simulink model "Drivetrain"  (R2013a)
settings: Solver=FixedStepDiscrete  StartTime=0.0  StopTime=10.0  FixedStep=.001  RelTol=1e-3
undefined symbols (not defined in the file or in its folder): power_lim, torque_lim
libraries: fl_lib x10, nesl_utility x6, sdl_lib x3, simulink x1
settings Model: Creator=noah  LastModifiedBy=ntfox
settings DataIOCC: SignalLoggingSaveFormat=ModelDataLogs
settings DebuggingCC: UnderspecifiedInitializationDetection=Simplified  MultiTaskDSMMsg=warning  MultiTaskCondExecSysMsg=none  StateNameClashWarn=none  StrictBusMsg=ErrorOnBusTreatedAsVector
settings RTWCC: IncludeERTFirstTime=on
settings GRTTargetCC: CodeReplacementLibrary=None  CPPClassGenCompliant=on

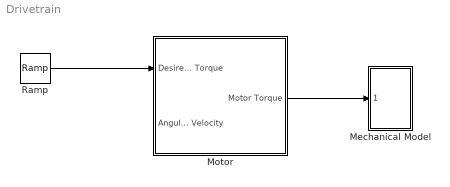
== system Drivetrain ==
  Mechanical Model : Subsystem
  Motor : Subsystem
  Ramp : simulink/Sources/Ramp  slope=1  start=0  X0=0
  wires:
  Motor/1(Motor Torque) -> Mechanical Model/1(Torque)
  Ramp/1 -> Motor/1(Desired Torque)

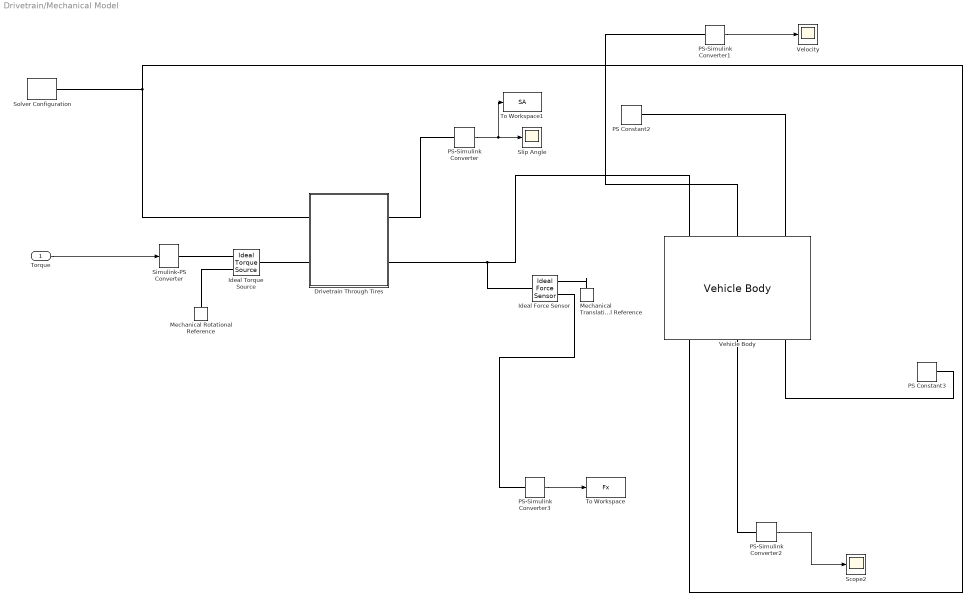
== system Drivetrain/Mechanical Model ==
  Torque : Inport
  Drivetrain Through Tires : Subsystem
  Ideal Force Sensor : fl_lib/Mechanical/Mechanical Sensors/Ideal Force Sensor  v_Log=off  f_Log=off  LocalVarNames=|v|f  LocalVarDescs=|v|f  LocalVarLogging=[0 0]
  Ideal Torque Source : fl_lib/Mechanical/Mechanical Sources/Ideal Torque Source  w_Log=off  t_Log=off  LocalVarNames=|w|t  LocalVarDescs=|w|t  LocalVarLogging=[0 0]
  Mechanical Rotational Reference : fl_lib/Mechanical/Rotational Elements/Mechanical Rotational Reference  t_Log=off  LocalVarNames=|t  LocalVarDescs=|t  LocalVarLogging=0
  Mechanical Translational Reference : fl_lib/Mechanical/Translational Elements/Mechanical Translational Reference  f_Log=off  LocalVarNames=|f  LocalVarDescs=|f  LocalVarLogging=0
  PS Constant2 : fl_lib/Physical Signals/Sources/PS Constant  constant=0  LocalVarLogging=[]
  PS Constant3 : fl_lib/Physical Signals/Sources/PS Constant  constant=0  LocalVarLogging=[]
  PS-Simulink Converter{,1..3} (4 alike) : nesl_utility/PS-Simulink Converter  PhysicalDomain=network_engine_domain  SubClassName=ps_output  LeftPortType=input  RightPortType=output  PseudoPeriodic=off  Frequencies=[]  Unit=1  AffineConversion=off
  Scope2 : Scope
      settings: SaveName=ScopeData2
  Simulink-PS Converter : nesl_utility/Simulink-PS Converter  PhysicalDomain=network_engine_domain  SubClassName=ps_input  LeftPortType=input  RightPortType=output  PseudoPeriodic=off  Frequencies=[]  NoiseDistribution=none  NoiseParameters=[]  Unit=1  AffineConversion=off  InputFiltering=off  SimscapeFilterOrder=1  InputFilterTimeConstant=0.001  UdotUserProvided=1
  Slip Angle : Scope
      settings: TimeRange=10  YMin=0  YMax=9000
  Solver Configuration : nesl_utility/Solver Configuration  PhysicalDomain=network_engine_domain  SubClassName=solver  LeftPortType=input  RightPortType=generic  Accelerate=off  Tones=[]  Harmonics=[]  SimulateNoise=off  Profile=off  UseLocalSampling=off  EnableSwitchedLinearOptims=on  FrequencyDomain=off  UseCCode=off  UseNewInitialization=off  DoDC=off  ResidualTolerance=1e-09  UseLocalSolver=off  LocalSolverChoice=NE_BACKWARD_EULER_ADVANCER  LocalSolverSampleTime=0.001  DoFixedCost=off  MaxNonlinIter=3  MaxModeIter=2  LinearAlgebra=Sparse  DelaysMemoryBudget=1024
  To Workspace : ToWorkspace  VariableName=Fx  SampleTime=-1  SaveFormat=Timeseries
  To Workspace1 : ToWorkspace  VariableName=SA  SampleTime=-1  SaveFormat=Timeseries
  Vehicle Body : sdl_lib/Tires & Vehicles/Vehicle Body  mass=300 kg  n_w=2  x_f=.8 m  x_r=.8 m  y_c=.2 m  area=3 m^2  Cd=0.4  v0=0 m/s  g=9.81 m/s^2  rho=1.18 kg/m^3  v_Log=off  f_Log=off  LocalVarNames=|v|f  LocalVarDescs=|v|f  LocalVarLogging=[0 0]
  Velocity : Scope
      settings: TimeRange=10  YMin=0  YMax=6
  wires:
  PS-Simulink Converter/1 -> To Workspace1/1, Slip Angle/1
  PS-Simulink Converter1/1 -> Velocity/1
  PS-Simulink Converter2/1 -> Scope2/1
  PS-Simulink Converter3/1 -> To Workspace/1
  Torque/1 -> Simulink-PS Converter/1
  connections:
  Simulink-PS Converter/RConn1 -- Ideal Torque Source/RConn1
  Mechanical Rotational Reference/LConn1 -- Ideal Torque Source/RConn2
  Drivetrain Through Tires/LConn2 -- Ideal Torque Source/LConn1
  PS-Simulink Converter/LConn1 -- Drivetrain Through Tires/RConn1
  Vehicle Body/RConn1 -- Drivetrain Through Tires/LConn1 -- Solver Configuration/RConn1
  Vehicle Body/RConn2 -- PS-Simulink Converter2/LConn1
  PS Constant2/RConn1 -- Vehicle Body/LConn3
  Vehicle Body/LConn2 -- PS-Simulink Converter1/LConn1
  PS Constant3/RConn1 -- Vehicle Body/RConn3
  Ideal Force Sensor/RConn2 -- PS-Simulink Converter3/LConn1
  Mechanical Translational Reference/LConn1 -- Ideal Force Sensor/RConn1
  Vehicle Body/LConn1 -- Ideal Force Sensor/LConn1 -- Drivetrain Through Tires/RConn2

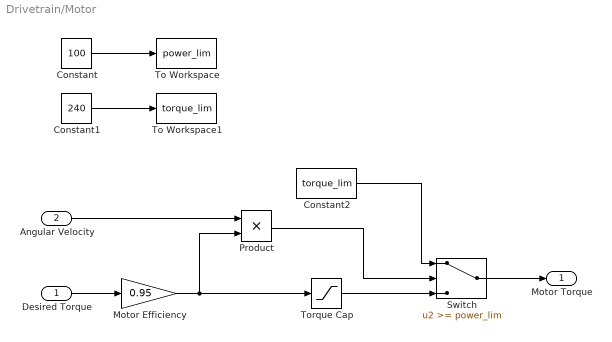
== system Drivetrain/Motor ==
  Desired Torque : Inport
  Angular Velocity : Inport  Port=2
  Constant : Constant  Value=100
  Constant1 : Constant  Value=240
  Constant2 : Constant  Value=torque_lim
  Motor Efficiency : Gain  Gain=0.95
  Product : Product
  Switch : Switch  Threshold=power_lim
  To Workspace : ToWorkspace  VariableName=power_lim  SampleTime=-1  SaveFormat=Timeseries
  To Workspace1 : ToWorkspace  VariableName=torque_lim  SampleTime=-1  SaveFormat=Timeseries
  Torque Cap : Saturate  UpperLimit=torque_lim  LowerLimit=-1*torque_lim
  Motor Torque : Outport
  wires:
  Switch/1 -> Motor Torque/1
  Torque Cap/1 -> Switch/3
  Constant1/1 -> To Workspace1/1
  Constant/1 -> To Workspace/1
  Desired Torque/1 -> Motor Efficiency/1
  Motor Efficiency/1 -> Product/2, Torque Cap/1
  Product/1 -> Switch/2
  Angular Velocity/1 -> Product/1
  Constant2/1 -> Switch/1

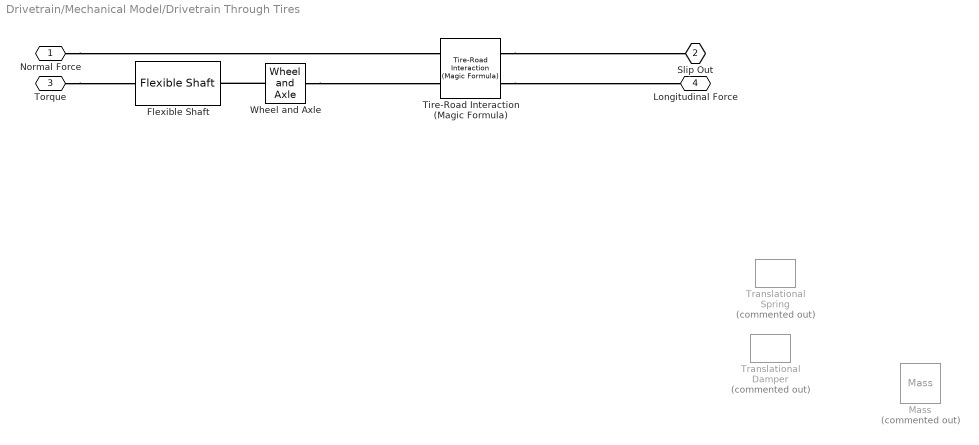
== system Drivetrain/Mechanical Model/Drivetrain Through Tires ==
  Flexible Shaft : sdl_lib/Couplings & Drives/Flexible Shaft  parameterization=1  shaft_stiffness=2e+50 N*m/rad  shaft_inertia=0.02 kg*m^2  shaft_construction=1  length=1 m  diameter_outer=0.075 m  diameter_inner=0.05 m  density=7.8e+3 kg/m^3  shear_modulus=7.93e+10 Pa  damping_ratio=0.01  n_segments=1  mu_visc=[ 0 0 ] N*m/(rad/s)  initial_deflection=0 rad  initial_velocity=0 rpm  LocalVarLogging=[]
  Mass : fl_lib/Mechanical/Translational Elements/Mass  Commented=on  mass=1 kg  initial_velocity=0 m/s  f_Log=off  LocalVarNames=|f  LocalVarDescs=|f  LocalVarLogging=0
  Tire-Road Interaction (Magic Formula) : sdl_lib/Tires & Vehicles/Tire Subcomponents/Tire-Road Interaction (Magic Formula)  parameterization=2  F_z1=3e+1 N  F_x1=3.5e+3 N  kappa1=10  B_m=10  C_m=1.9  D_m=1  E_m=0.97  fz0=4e+3 N  p_Cx=1.685  p_Dx=[ 1.21 -0.037 ]  p_Ex=[ 0.344 0.095 -0.02 0 ]  p_Kx=[ 21.51 -0.163 0.245 ]  p_Hx=[ -0.002 0.002 ]  p_Vx=[ 0 0 ]  v_tr_thr=0.1 m/s  LocalVarLogging=[]
  Translational Damper : fl_lib/Mechanical/Translational Elements/Translational Damper  Commented=on  D=100 N/(m/s)  f_Log=off  v_Log=off  LocalVarNames=|f|v  LocalVarDescs=|f|v  LocalVarLogging=[0 0]
  Translational Spring : fl_lib/Mechanical/Translational Elements/Translational Spring  Commented=on  spr_rate=1000 N/m  init_def=0 m  f_Log=off  v_Log=off  x_Log=off  LocalVarNames=|f|v|x  LocalVarDescs=|f|v|x  LocalVarLogging=[0 0 0]
  Wheel and Axle : fl_lib/Mechanical/Mechanisms/Wheel and Axle  R=.2 m  or=1  orient=1  t_Log=off  f_Log=off  LocalVarNames=|t|f  LocalVarDescs=|t|f  LocalVarLogging=[0 0]
  Normal Force : PMIOPort  Port=1  Side=Left
  Slip Out : PMIOPort  Port=2  Side=Right
  Torque : PMIOPort  Port=3  Side=Left
  Longitudinal Force : PMIOPort  Port=4  Side=Right
  connections:
  Tire-Road Interaction (Magic Formula)/RConn2 -- Longitudinal Force/RConn1
  Tire-Road Interaction (Magic Formula)/RConn1 -- Slip Out/RConn1
  Normal Force/RConn1 -- Tire-Road Interaction (Magic Formula)/LConn1
  Wheel and Axle/RConn1 -- Tire-Road Interaction (Magic Formula)/LConn2
  Wheel and Axle/LConn1 -- Flexible Shaft/RConn1
  Torque/RConn1 -- Flexible Shaft/LConn1
